simulink model "TuneWall"  (R2025b)
settings: Solver=VariableStepAuto  StartTime=0.0  StopTime=3600*4  RelTol=1e-3
model workspace (MAT data in the model file):
  h_in = 1.419
  h_out = 3.859
  k_Block = 0.01
  k_concrete = 0.11
libraries: fl_lib x66, nesl_utility x19, SimscapeFluids_lib x8
(part 1 of 2)
settings Model: Creator=Windows  LastModifiedBy=acer

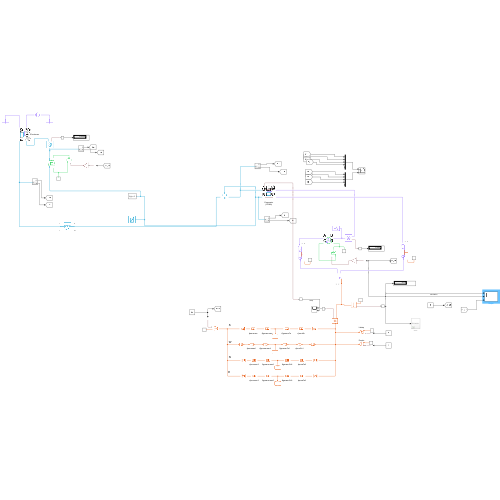
[thumbnail: Simulink's stored preview of the top-level diagram]
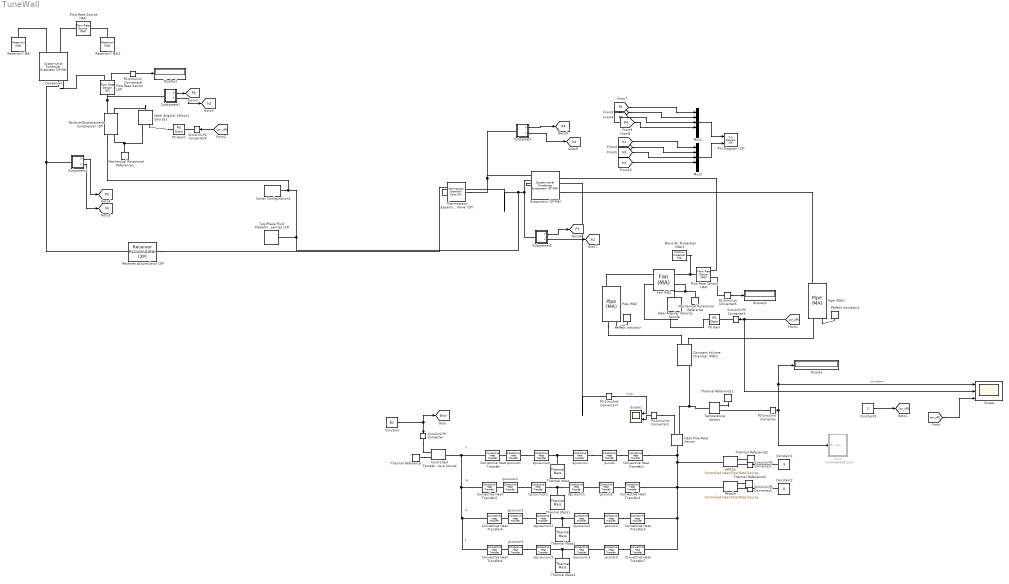
== system TuneWall ==
  note: S
  note: W
  note: N
  note: E
  Condenser : SimscapeFluids_lib/Heat Exchangers/Two-Phase Fluid - Moist Air/System-Level Condenser Evaporator (2P-MA)  flow_arrangement=fluids.heat_exchangers.enum.SystemLevelFlowArrangement2PMA.Counter  wall_thermal_mass=false  mass_wall=1 kg  cp_wall=490 J/(K*kg)  nominal_init_wall=true  T_wall_init=293.15 K  area_A1=0.01 m^2  area_B1=0.01 m^2  area_A2=0.01 m^2  area_B2=0.01 m^2  operating_condition_2P=fluids.heat_exchangers.enum.SystemLevelOperatingCondition2PMA.Condenser  mdot_nominal_2P=0.0142 kg/s  delta_p_nominal_2P=0.01 MPa  pressure_spec_cond_2P=fluids.heat_exchangers.enum.SystemLevelPressureSpecCondenser2P.InletPressure  pressure_spec_evap_2P=fluids.heat_exchangers.enum.SystemLevelPressureSpecEvaporator2P.InletPressure  p_in_nominal_2P=1.673 MPa  T_cond_nominal_2P=313.15 K  T_evap_nominal_2P=243.15 K  inlet_spec_2P=fluids.heat_exchangers.enum.SystemLevelInletSpec2P.Enthalpy  T_in_nominal_2P=333.15 K  h_in_nominal_2P=423.9 kJ/kg  x_in_nominal_2P=1  capacity_spec_2P=fluids.heat_exchangers.enum.SystemLevelCapacitySpec.HeatTransfer  Q_nominal=2.404 kW  outlet_spec_cond_2P=fluids.heat_exchangers.enum.SystemLevelOutletSpecCondenser2P.Enthalpy  outlet_spec_evap_2P=fluids.heat_exchangers.enum.SystemLevelOutletSpecEvaporator2P.Enthalpy  delta_T_sub_nominal_2P=5 deltaK  delta_T_sup_nominal_2P=5 deltaK  h_out_nominal_2P=250 kJ/kg  x_out_nominal_2P=0  volume_2P=0.001 m^3  nominal_init_2P=true  energy_spec_2P=foundation.enum.energy_spec.enthalpy  p_init_2P=0.101325 MPa  T_init_2P=293.15 K  x_init_2P=0.5  alpha_init_2P=0.5  h_init_2P=1500 kJ/kg  u_init_2P=1500 kJ/kg  mdot_nominal_MA=1 kg/s  delta_p_nominal_MA=0.001 MPa  p_in_nominal_MA=0.101325 MPa  T_in_nominal_MA=293.15 K  inlet_humidity_spec_MA=foundation.enum.HumiditySpec.RelativeHumidity  RH_in_nominal_MA=0.5  x_w_in_nominal_MA=0.01  y_w_in_nominal_MA=0.01  HR_in_nominal_MA=0.01  Tw_in_nominal_MA=287 K  inlet_trace_gas_spec_MA=foundation.enum.trace_gas_spec.mass_fraction  x_g_in_nominal_MA=0.001  y_g_in_nominal_MA=0.001  volume_MA=0.1 m^3  nominal_init_MA=true  p_init_MA=0.101325 MPa  T_init_MA=293.15 K  humidity_spec_MA=foundation.enum.HumiditySpec.RelativeHumidity  RH_init_MA=0.5  x_w_init_MA=0.01  y_w_init_MA=0.01  HR_init_MA=0.01  Tw_init_MA=287 K  trace_gas_spec_MA=foundation.enum.trace_gas_spec.mass_fraction  x_g_init_MA=0.001  y_g_init_MA=0.001  r_d_init_MA=0  RH_ws_MA=1  time_constant_cond_MA=1e-3 s  time_constant_evap_MA=1e-3 s  fraction_entrained_MA=1  a_liq_2P=0.023  a_mix_2P=0.005  a_vap_2P=0.023  b_2P=0.8  c_2P=0.33  a_MA=0.023  b_MA=0.8  c_MA=0.33
      settings: InternalSimscapePortConfiguration="{\"Bottom\":[],\"Left\":[{\"id\":\"A1\",\"label\":\"A1\",\"type\":\"foundation.two_phase_fluid.two_phase_fluid\"},{\"id\":\"B1\",\"label\":\"B1\",\"type\":\"foundation.two_phase_fluid.two_phase_fluid\"}],\"Right\":[{\"id\":\"A2\",\"label\":\"A2\",\"type\":\"foundation.moist_air.moist_air\"},{\"id\":\"B2\",\"label\":\"B2\",\"type\":\"foundation.moist_air.moist_air\"}],\"Top\":[{\"id\":\"Q1\",\"label\":\"Q1\",\"type\":\"output\"},{\"id\":\"Q2\",\"label\":\"Q2\",\"type\":\"output\"},{\"id\":\"W\",\"label\":\"W\",\"type\":\"output\"}]}"
  Constant : Constant  Value=30
  Constant Volume Chamber (MA)2 : fl_lib/Moist Air/Elements/Constant Volume Chamber (MA)  volume=92.924 m^3  num_ports=foundation.enum.num_ports.two  area_A=0.01 m^2  area_B=0.01 m^2  area_C=0.01 m^2  area_D=0.01 m^2  RH_ws=1  time_constant_cond=1e-3 s  time_constant_evap=1e-3 s  fraction_entrained=1  moisture_trace_gas_source=foundation.enum.moisture_trace_gas_source.none  moisture_source_spec=foundation.enum.MoistureSourceSpec.WaterVapor  vapor_from_liquid=false  moisture_mass_flow=0 kg/s  moisture_temperature_spec=foundation.enum.temperature_spec.atmospheric  moisture_temperature=293.15 K  trace_gas_mass_flow=0 kg/s  trace_gas_temperature_spec=foundation.enum.temperature_spec.atmospheric  trace_gas_temperature=293.15 K  p_init=0.101325 MPa  p_init_priority=foundation.enum.Priority.High  T_init=273.15+30 K  T_init_priority=foundation.enum.Priority.High  humidity_spec=foundation.enum.HumiditySpec.RelativeHumidity  RH_init=0.6  RH_init_priority=foundation.enum.Priority.High  x_w_init=0.01  x_w_init_priority=foundation.enum.Priority.High  y_w_init=0.01  y_w_init_priority=foundation.enum.Priority.High  HR_init=0.01  HR_init_priority=foundation.enum.Priority.High  Tw_init=287 K  Tw_init_priority=foundation.enum.Priority.High  trace_gas_spec=foundation.enum.trace_gas_spec.mass_fraction  x_g_init=0.001  x_g_init_priority=foundation.enum.Priority.High  y_g_init=0.001  y_g_init_priority=foundation.enum.Priority.High  r_d_init=0  r_d_init_priority=foundation.enum.Priority.High
      settings: InternalSimscapePortConfiguration="{\"Bottom\":[],\"Left\":[{\"id\":\"A\",\"label\":\"A\",\"type\":\"foundation.moist_air.moist_air\"},{\"id\":\"B\",\"label\":\"B\",\"type\":\"foundation.moist_air.moist_air\"}],\"Right\":[{\"id\":\"W\",\"label\":\"W\",\"type\":\"output\"},{\"id\":\"F\",\"label\":\"F\",\"type\":\"output\"},{\"id\":\"H\",\"label\":\"H\",\"type\":\"foundation.thermal.thermal\"}],\"Top\":[]}"
  Constant1 : Constant  Value=3
  Constant2 : Constant  Value=0
  Constant3 : Constant
  Controlled Temperature Source : fl_lib/Thermal/Thermal Sources/Controlled Temperature Source
  Convective Heat Transfer : fl_lib/Thermal/Thermal Elements/Convective Heat Transfer  thermal_type=foundation.enum.constant_variable.constant  area=8.51*3 m^2  heat_tr_coeff=h_out W/(K*m^2)  min_heat_tr_coeff=1e-3 W/(K*m^2)  T_specify=off  T_priority=None  T=0 K  T_nominal_specify=off  T_nominal_value=1  T_nominal_unit=K  Q_specify=off  Q_priority=None  Q=0 W  Q_nominal_specify=off  Q_nominal_value=1  Q_nominal_unit=W
  Convective Heat Transfer1 : fl_lib/Thermal/Thermal Elements/Convective Heat Transfer  thermal_type=foundation.enum.constant_variable.constant  area=8.51*3 m^2  heat_tr_coeff=h_in W/(K*m^2)  min_heat_tr_coeff=1e-3 W/(K*m^2)  T_specify=off  T_priority=None  T=0 K  T_nominal_specify=off  T_nominal_value=1  T_nominal_unit=K  Q_specify=off  Q_priority=None  Q=0 W  Q_nominal_specify=off  Q_nominal_value=1  Q_nominal_unit=W
  Convective Heat Transfer2 : fl_lib/Thermal/Thermal Elements/Convective Heat Transfer  thermal_type=foundation.enum.constant_variable.constant  area=8.86*3 m^2  heat_tr_coeff=h_out W/(K*m^2)  min_heat_tr_coeff=1e-3 W/(K*m^2)  T_specify=off  T_priority=None  T=0 K  T_nominal_specify=off  T_nominal_value=1  T_nominal_unit=K  Q_specify=off  Q_priority=None  Q=0 W  Q_nominal_specify=off  Q_nominal_value=1  Q_nominal_unit=W
  Convective Heat Transfer3 : fl_lib/Thermal/Thermal Elements/Convective Heat Transfer  thermal_type=foundation.enum.constant_variable.constant  area=8.86*3 m^2  heat_tr_coeff=h_in W/(K*m^2)  min_heat_tr_coeff=1e-3 W/(K*m^2)  T_specify=off  T_priority=None  T=0 K  T_nominal_specify=off  T_nominal_value=1  T_nominal_unit=K  Q_specify=off  Q_priority=None  Q=0 W  Q_nominal_specify=off  Q_nominal_value=1  Q_nominal_unit=W
  Convective Heat Transfer4 : fl_lib/Thermal/Thermal Elements/Convective Heat Transfer  thermal_type=foundation.enum.constant_variable.constant  area=8.51*3 m^2  heat_tr_coeff=h_out W/(K*m^2)  min_heat_tr_coeff=1e-3 W/(K*m^2)  T_specify=off  T_priority=None  T=0 K  T_nominal_specify=off  T_nominal_value=1  T_nominal_unit=K  Q_specify=off  Q_priority=None  Q=0 W  Q_nominal_specify=off  Q_nominal_value=1  Q_nominal_unit=W
  Convective Heat Transfer5 : fl_lib/Thermal/Thermal Elements/Convective Heat Transfer  thermal_type=foundation.enum.constant_variable.constant  area=8.51*3 m^2  heat_tr_coeff=h_in W/(K*m^2)  min_heat_tr_coeff=1e-3 W/(K*m^2)  T_specify=off  T_priority=None  T=0 K  T_nominal_specify=off  T_nominal_value=1  T_nominal_unit=K  Q_specify=off  Q_priority=None  Q=0 W  Q_nominal_specify=off  Q_nominal_value=1  Q_nominal_unit=W
  Convective Heat Transfer6 : fl_lib/Thermal/Thermal Elements/Convective Heat Transfer  thermal_type=foundation.enum.constant_variable.constant  area=8.86*3 m^2  heat_tr_coeff=h_out W/(K*m^2)  min_heat_tr_coeff=1e-3 W/(K*m^2)  T_specify=off  T_priority=None  T=0 K  T_nominal_specify=off  T_nominal_value=1  T_nominal_unit=K  Q_specify=off  Q_priority=None  Q=0 W  Q_nominal_specify=off  Q_nominal_value=1  Q_nominal_unit=W
  Convective Heat Transfer7 : fl_lib/Thermal/Thermal Elements/Convective Heat Transfer  thermal_type=foundation.enum.constant_variable.constant  area=8.86*3 m^2  heat_tr_coeff=h_in W/(K*m^2)  min_heat_tr_coeff=1e-3 W/(K*m^2)  T_specify=off  T_priority=None  T=0 K  T_nominal_specify=off  T_nominal_value=1  T_nominal_unit=K  Q_specify=off  Q_priority=None  Q=0 W  Q_nominal_specify=off  Q_nominal_value=1  Q_nominal_unit=W
  Display : Display
      settings: Decimation=3
  Display1 : Display
  Display2 : Display
  Evaporator (2P-MA) : SimscapeFluids_lib/Heat Exchangers/Two-Phase Fluid - Moist Air/System-Level Condenser Evaporator (2P-MA)  flow_arrangement=fluids.heat_exchangers.enum.SystemLevelFlowArrangement2PMA.Counter  wall_thermal_mass=false  mass_wall=1 kg  cp_wall=490 J/(K*kg)  nominal_init_wall=true  T_wall_init=293.15 K  area_A1=0.71 cm^2  area_B1=1.96 cm^2  area_A2=0.01 m^2  area_B2=0.01 m^2  operating_condition_2P=fluids.heat_exchangers.enum.SystemLevelOperatingCondition2PMA.Evaporator  mdot_nominal_2P=0.0142 kg/s  delta_p_nominal_2P=0.01 MPa  pressure_spec_cond_2P=fluids.heat_exchangers.enum.SystemLevelPressureSpecCondenser2P.InletPressure  pressure_spec_evap_2P=fluids.heat_exchangers.enum.SystemLevelPressureSpecEvaporator2P.InletPressure  p_in_nominal_2P=0.5806 MPa  T_cond_nominal_2P=313.15 K  T_evap_nominal_2P=243.15 K  inlet_spec_2P=fluids.heat_exchangers.enum.SystemLevelInletSpec2P.Enthalpy  T_in_nominal_2P=333.15 K  h_in_nominal_2P=253.3 kJ/kg  x_in_nominal_2P=1  capacity_spec_2P=fluids.heat_exchangers.enum.SystemLevelCapacitySpec.HeatTransfer  Q_nominal=2.31 kW  outlet_spec_cond_2P=fluids.heat_exchangers.enum.SystemLevelOutletSpecCondenser2P.Enthalpy  outlet_spec_evap_2P=fluids.heat_exchangers.enum.SystemLevelOutletSpecEvaporator2P.Enthalpy  delta_T_sub_nominal_2P=5 deltaK  delta_T_sup_nominal_2P=5 deltaK  h_out_nominal_2P=250 kJ/kg  x_out_nominal_2P=0  volume_2P=0.001 m^3  nominal_init_2P=true  energy_spec_2P=foundation.enum.energy_spec.enthalpy  p_init_2P=0.101325 MPa  T_init_2P=293.15 K  x_init_2P=0.5  alpha_init_2P=0.5  h_init_2P=1500 kJ/kg  u_init_2P=1500 kJ/kg  mdot_nominal_MA=1 kg/s  delta_p_nominal_MA=0.001 MPa  p_in_nominal_MA=0.101325 MPa  T_in_nominal_MA=29+273.15 K  inlet_humidity_spec_MA=foundation.enum.HumiditySpec.RelativeHumidity  RH_in_nominal_MA=0.5  x_w_in_nominal_MA=0.01  y_w_in_nominal_MA=0.01  HR_in_nominal_MA=0.01  Tw_in_nominal_MA=287 K  inlet_trace_gas_spec_MA=foundation.enum.trace_gas_spec.mass_fraction  x_g_in_nominal_MA=0.001  y_g_in_nominal_MA=0.001  volume_MA=0.1 m^3  nominal_init_MA=true  p_init_MA=0.101325 MPa  T_init_MA=293.15 K  humidity_spec_MA=foundation.enum.HumiditySpec.RelativeHumidity  RH_init_MA=0.5  x_w_init_MA=0.01  y_w_init_MA=0.01  HR_init_MA=0.01  Tw_init_MA=287 K  trace_gas_spec_MA=foundation.enum.trace_gas_spec.mass_fraction  x_g_init_MA=0.001  y_g_init_MA=0.001  r_d_init_MA=0  RH_ws_MA=1  time_constant_cond_MA=1e-3 s  time_constant_evap_MA=1e-3 s  fraction_entrained_MA=1  a_liq_2P=0.023  a_mix_2P=0.005  a_vap_2P=0.023  b_2P=0.8  c_2P=0.33  a_MA=0.023  b_MA=0.8  c_MA=0.33
      settings: InternalSimscapePortConfiguration="{\"Bottom\":[],\"Left\":[{\"id\":\"A1\",\"label\":\"A1\",\"type\":\"foundation.two_phase_fluid.two_phase_fluid\"},{\"id\":\"B1\",\"label\":\"B1\",\"type\":\"foundation.two_phase_fluid.two_phase_fluid\"}],\"Right\":[{\"id\":\"A2\",\"label\":\"A2\",\"type\":\"foundation.moist_air.moist_air\"},{\"id\":\"B2\",\"label\":\"B2\",\"type\":\"foundation.moist_air.moist_air\"}],\"Top\":[{\"id\":\"Q1\",\"label\":\"Q1\",\"type\":\"output\"},{\"id\":\"Q2\",\"label\":\"Q2\",\"type\":\"output\"},{\"id\":\"W\",\"label\":\"W\",\"type\":\"output\"}]}"
  Fan (MA) : SimscapeFluids_lib/Moist Air/Turbomachinery/Fan (MA)  fan_parameterization=fluids.moist_air.turbomachinery.enum.FanParameterization.Nominal  mechanical_power_spec=fluids.moist_air.turbomachinery.enum.FanMechanicalPowerSpec.Efficiency  flow_rate_nominal=0.38 m^3/s  pressure_nominal=5400 Pa  eta_nominal=1  power_nominal=1620 W  pressure_max=6400 Pa  flow_rate_max=0.4 m^3/s  omega_ref_nominal=1800 rpm  flow_rate_1D_TLU=[.0278, .0556, .0833, .111, .139, .167] m^3/s  pressure_1D_TLU=[6410, 6375, 6018, 5366, 4501, 3609] Pa  eta_1D_TLU=[.257, .394, .453, .47, .459, .415]  power_1D_TLU=[693, 900, 1107, 1267, 1363, 1452] W  omega_ref_1D=3000 rpm  rho_ref_1D=1.2 kg/m^3  omega_threshold_factor=1e-2  omega_dp_TLU=[2400; 3000; 3600] rpm  flow_rate_dp_TLU=[.0278, .0556, .0833, .111, .139, .167] m^3/s  pressure_dp_TLU=[4111, 4010, 3551, 2881, 2167, 1453; 6410, 6375, 6018, 5366, 4501, 3609; 9217, 9285, 9022, 8428, 7552, 6482] Pa  eta_dp_TLU=[.3, .434, .468, .459, .4, .3; .257, .394, .453, .47, .459, .415; .225, .359, .434, .461, .47, .459]  power_dp_TLU=[381, 514, 632, 697, 753, 809; 693, 900, 1107, 1267, 1363, 1452; 1139, 1438, 1732, 2029, 2233, 2358] W  rho_ref_dp=1.2 kg/m^3  omega_q_TLU=[2990; 3450; 3867] rpm  pressure_q_TLU=[31, 62, 93, 124] Pa  flow_rate_q_TLU=[.802, .759, .703, .611; .936, .902, .862, .81; 1.056, 1.027, .994, .956] m^3/s  eta_q_TLU=[.088, .162, .22, .261; .068, .128, .18, .222; .055, .105, .148, .188]  power_q_TLU=[283, 290, 297, 290; 427, 437, 445, 452; 595, 606, 625, 631] W  rho_ref_q=1.2 kg/m^3  diameter_ratio=1  mech_orientation=fluids.moist_air.turbomachinery.enum.FanMechanicalOrientation.Positive  area_A=0.01 m^2  area_B=0.01 m^2
      settings: InternalSimscapePortConfiguration="{\"Bottom\":[],\"Left\":[{\"id\":\"A\",\"label\":\"A\",\"type\":\"foundation.moist_air.moist_air\"},{\"id\":\"C\",\"label\":\"C\",\"type\":\"foundation.mechanical.rotational.rotational\"}],\"Right\":[{\"id\":\"B\",\"label\":\"B\",\"type\":\"foundation.moist_air.moist_air\"},{\"id\":\"R\",\"label\":\"R\",\"type\":\"foundation.mechanical.rotational.rotational\"}],\"Top\":[]}"
  Flow Rate Sensor (2P) : fl_lib/Two-Phase Fluid/Sensors/Flow Rate Sensor (2P)  mass_flow_measure=true  volumetric_flow_measure=false  energy_flow_measure=false
      settings: InternalSimscapePortConfiguration="{\"Bottom\":[],\"Left\":[{\"id\":\"A\",\"label\":\"A\",\"type\":\"foundation.two_phase_fluid.two_phase_fluid\"}],\"Right\":[{\"id\":\"B\",\"label\":\"B\",\"type\":\"foundation.two_phase_fluid.two_phase_fluid\"},{\"id\":\"M\",\"label\":\"M\",\"type\":\"output\"}],\"Top\":[]}"
  Flow Rate Sensor (MA) : fl_lib/Moist Air/Sensors/Flow Rate Sensor (MA)  mass_flow_measure=true  volumetric_flow_measure=false  volumetric_flow_conditions=foundation.enum.volumetric_flow_conditions.actual  p_std=0.101325 MPa  T_std=20 degC  RH_std=0.65  energy_flow_measure=false  vapor_flow_measure=false  gas_flow_measure=false  droplets_flow_measure=false
      settings: InternalSimscapePortConfiguration="{\"Bottom\":[],\"Left\":[{\"id\":\"A\",\"label\":\"A\",\"type\":\"foundation.moist_air.moist_air\"}],\"Right\":[{\"id\":\"B\",\"label\":\"B\",\"type\":\"foundation.moist_air.moist_air\"},{\"id\":\"M\",\"label\":\"M\",\"type\":\"output\"}],\"Top\":[]}"
  Flow Rate Source (MA) : fl_lib/Moist Air/Sources/Flow Rate Source (MA)  source_type=foundation.enum.constant_controlled.constant  flow_type=foundation.enum.mass_volumetric_flow.mass  mass_flow=1 kg/s  volumetric_flow=0 m^3/s  volumetric_flow_conditions=foundation.enum.volumetric_flow_conditions.actual  p_std=0.101325 MPa  T_std=20 degC  RH_std=0.65  power_spec=foundation.enum.power_spec.isentropic  area_A=0.01 m^2  area_B=0.01 m^2
      settings: InternalSimscapePortConfiguration="{\"Bottom\":[],\"Left\":[{\"id\":\"A\",\"label\":\"A\",\"type\":\"foundation.moist_air.moist_air\"}],\"Right\":[{\"id\":\"B\",\"label\":\"B\",\"type\":\"foundation.moist_air.moist_air\"}],\"Top\":[]}"
  Heat Flow Rate Sensor : fl_lib/Thermal/Thermal Sensors/Heat Flow Rate Sensor
  Ideal Angular Velocity Source : fl_lib/Mechanical/Mechanical Sources/Ideal Angular Velocity Source
  Ideal Angular Velocity Source1 : fl_lib/Mechanical/Mechanical Sources/Ideal Angular Velocity Source
  Labtop : fl_lib/Thermal/Thermal Sources/Controlled Heat Flow Rate Source
  Mechanical Rotational Reference : fl_lib/Mechanical/Rotational Elements/Mechanical Rotational Reference
  Mechanical Rotational Reference1 : fl_lib/Mechanical/Rotational Elements/Mechanical Rotational Reference
  Moist Air Properties (MA)1 : fl_lib/Moist Air/Utilities/Moist Air Properties (MA)  R_a=287.047 J/(K*kg)  T_TLU=[-56.55, -50 : 10 : -10, -5 : 1 : 5, 10 : 10 : 350]' degC  h_a_TLU=[342.414066793634; 349.003411914139; 359.061417476782; 369.117728274935; 379.173188407993; 389.228602960013; 394.256538873206; 395.262156814682; 396.26778682262; 397.27342967397; 398.279086145689; 399.284757014822; 400.290443058569; 401.296145054364; 402.301863779931; 403.307600013352; 404.313354533128; 409.342428711098; 419.402397945314; 429.465451846544; 439.532387826623; 449.604014793745; 459.68115297076; 469.764632657687; 479.855292205971; 489.953975419749; 500.06152856014; 510.178797098051; 520.306622336267; 530.445838000969; 540.597266885076; 550.761717610289; 560.939981561004; 571.132830031086; 581.341011613777; 591.565249855533; 601.806241186423; 612.064653132654; 622.341122810862; 632.636255698901; 642.95062467384; 653.284769304793; 663.639195385783; 674.014374692179; 684.410744943084; 694.828709951456; 705.268639943519; 715.730872029167; 726.215710805484; 736.723429076127; 747.254268670154; 757.808441344776] kJ/kg  mu_a_TLU=[14.2568884161326; 14.6140128551699; 15.151727785151; 15.6806860927178; 16.201235181264; 16.7137043838401; 16.9670072430524; 17.017438132541; 17.0677931537044; 17.1180726001803; 17.1682767640582; 17.2184059358881; 17.2684604046898; 17.318440457962; 17.3683463816913; 17.4181784603614; 17.467936976962; 17.7156359301048; 18.2056752419787; 18.6887904184394; 19.1652345249932; 19.6352479488881; 20.099059157425; 20.5568854116507; 21.008933436444; 21.4554000485251; 21.8964727442509; 22.3323302492491; 22.7631430320408; 23.1890737838183; 23.6102778665211; 24.0269037312887; 24.4390933092858; 24.8469823767971; 25.2507008963847; 25.6503733357905; 26.0461189661617; 26.438052141067; 26.8262825576728; 27.210915501349; 27.5920520748824; 27.969789413389; 28.3442208859359; 28.7154362848061; 29.0835220032714; 29.4485612026716; 29.8106339695395; 30.169817463453; 30.5261860562487; 30.8798114631771; 31.2307628665438; 31.5791070323335] s*uPa  k_a_TLU=[19.8808491891482; 20.4162457047568; 21.2248745869044; 22.0232455041378; 22.8117316528767; 23.59069155438; 23.9767077285082; 24.0536401764626; 24.130482853517; 24.2072360894785; 24.2839002127411; 24.3604755502875; 24.4369624276914; 24.5133611691197; 24.5896720973349; 24.6658955336975; 24.7420317981691; 25.1214166432482; 25.8738284673185; 26.6180151791963; 27.3542675863918; 28.0828636150405; 28.8040688184917; 29.5181369069754; 30.2253102842368; 30.9258205811167; 31.6198891790667; 32.307727718801; 32.989538590917; 33.6655154065126; 34.3358434467079; 35.0007000906151; 35.6602552217624; 36.314671613305; 36.9641052925838; 37.6087058857479; 38.2486169432557; 38.8839762471259; 39.5149161008418; 40.1415636028127; 40.7640409042923; 41.3824654526272; 41.9969502206863; 42.6076039232795; 43.2145312213471; 43.8178329146528; 44.4176061236819; 45.0139444614019; 45.6069381955058; 46.1966744017242; 46.7832371087507; 47.3667074352967] mW/(K*m)  p_min=1 kPa  p_max=inf MPa  T_min=-56.55 degC  T_max=350 degC  properties_range_check=simscape.enum.assert.action.error  p_atm=0.101325 MPa  T_atm=20 degC  enable_droplets=false  R_w=461.523 J/(K*kg)  p_ws_TLU=[1.71168953425982e-06; 3.93770601979424e-06; 1.28411717710344e-05; 3.80051394873809e-05; .00010323902900209; .000259873810798063; .000401741022116384; .000437454836117844; .000476040820618202; .000517704666185737; .000562664883741207; .000611212677444345; .000657085634113763; .000705985593917791; .00075808051438111; .000813548355379396; .000872575113841924; .00122819910164487; .00233931836947519; .00424697076171126; .00738493802968097; .012351945812707; .0199464343236764; .0312009300307261; .0474144740241604; .0701817658485933; .101417996663294; .143378712947169; .198674420476403; .270279976781692; .361539099388177; .476164537971214; .618234621423587; .792187006980199; 1.00281053608169; 1.25523615516845; 1.55492790046272; 1.90767499353199; 2.31958617020155; 2.79708749692822; 3.34692514426746; 3.97617493064794; 4.69226099229504; 5.50298678300951; 6.41658290952841; 7.44177834442093; 8.58790494083256; 9.86505121117553; 11.284292927457; 12.8580516000122; 14.6006773719404; 16.5294151389953] MPa  h_w_vap_TLU=[2836.88241275372; 2837.81392500514; 2838.63937175807; 2838.7309929628; 2838.06905313927; 2836.62597341095; 2835.60023952573; 2835.37006381376; 2835.13143158077; 2834.88429145066; 2834.62859062897; 2500.93420564316; 2498.55452890293; 2496.17317793437; 2493.7941260618; 2491.41713708944; 2489.04199020767; 2477.18706302224; 2453.51925941961; 2429.81122987564; 2405.97728678685; 2381.94712654051; 2357.65452030374; 2333.03120800924; 2308.00352809267; 2282.49062771796; 2256.40372152657; 2229.64615315163; 2202.11407337172; 2173.6974807639; 2144.28128268553; 2113.74600964951; 2081.9678834089; 2048.81807129851; 2014.16109962579; 1977.85249331179; 1939.73572816654; 1899.63852389863; 1857.36838273035; 1812.70710332357; 1765.4037880462; 1715.16561416478; 1661.64526339623; 1604.4232249434; 1542.98206457018; 1476.66790089115; 1404.63083498414; 1325.72875296442; 1238.36212284382; 1140.16281350074; 1027.31658328826; 892.746804215825] kJ/kg  h_w_TLU=[2396.53078650168; 2408.65722023252; 2427.16766028467; 2445.66624034104; 2464.1379798878; 2482.5594701893; 2491.7412703989; 2493.57467660537; 2495.40699233755; 2497.23816944599; 2499.06815833272; 2500.89261781717; 2502.73123919979; 2504.56496564907; 2506.39800457704; 2508.23033644628; 2510.06194120626; 2519.20831890725; 2537.43340437276; 2555.54520329515; 2573.51032237465; 2591.28888786817; 2608.83487221908; 2626.09640083333; 2643.01588134754; 2659.53001419864; 2675.5827869577; 2696.18462565746; 2716.49989554204; 2736.6235211014; 2756.61216047677; 2776.50561774616; 2796.33378923373; 2816.11979584021; 2835.88181424959; 2855.6343057571; 2875.38889328914; 2895.15500578618; 2914.94035966265; 2934.75132291939; 2954.59319332093; 2974.47041287496; 2994.38673461102; 3014.34535330297; 3034.34900869544; 3054.40006758361; 3074.50058949656; 3094.65237956705; 3114.85703131193; 3135.11596141057; 3155.43043809331; 3175.80160439414] kJ/kg  mu_w_TLU=[6.9886414857741; 7.21462000349698; 7.55962537406626; 7.90463074463554; 8.24963611520482; 8.5946414857741; 8.76714417105874; 8.80164470811567; 8.8361452451726; 8.87064578222952; 8.90514631928645; 8.93964685634338; 8.97414739340031; 9.00294911497154; 9.0318980288863; 9.06099135942002; 9.09022638806001; 9.23843559844524; 9.5440595677542; 9.86015858692705; 10.1848429274122; 10.5164578096049; 10.8535319382781; 11.1947482575333; 11.5389294976352; 11.8850331780701; 12.2322493177351; 12.6188533568459; 13.0082793358938; 13.4003380262893; 13.7948421428098; 14.1916095618232; 14.590464747099; 14.9912394314964; 15.3937729006119; 15.7979120385447; 16.203511226482; 16.610432150303; 17.0185435533718; 17.4277209582061; 17.8378463726577; 18.2488079909412; 18.6604998963166; 19.0728217698535; 19.485678608085; 19.8989804512625; 20.3126421231677; 20.7265829829225; 21.1407266888906; 21.5550009745266; 21.969337435876; 22.3836713303269] s*uPa  k_w_TLU=[12.4916816538045; 12.9847788176262; 13.737598915064; 14.4904190125018; 15.2432391099396; 15.9960592073774; 16.3724692560963; 16.4477512658401; 16.5230332755839; 16.5983152853277; 16.6735972950715; 16.7488793048152; 16.824161314559; 16.8886088206517; 16.9532779906513; 17.0181691764255; 17.083282769915; 17.4122036181723; 18.0870861656185; 18.7855813517187; 19.5093466408385; 20.2607864040347; 21.0430876297671; 21.8602068151121; 22.7168164077153; 23.6182141540994; 24.5698636875305; 25.4024944426483; 26.2458938647479; 27.1009155051916; 27.968142896353; 28.8479507975112; 29.7405485790829; 30.646029672269; 31.5643932662527; 32.4955693285114; 33.4394360046859; 34.3958329885356; 35.3645718140131; 36.3454437886179; 37.3382261129791; 38.3426866012072; 39.3585873185985; 40.3856873794121; 41.4237450915028; 42.4725195920623; 43.5317720862424; 44.6012667755489; 45.6807715437344; 46.7700584531355; 47.8689040929333; 48.9770898119082] mW/(K*m)  D_w=25 mm^2/s  trace_gas_model=foundation.enum.trace_gas_model.none  R_g=188.923 J/(K*kg)  h_g_TLU=[439.555216276024; 444.670268214299; 452.538618857965; 460.487124266174; 468.522588773143; 476.64941595933; 480.747985385885; 481.570543185868; 482.394052396612; 483.218514286302; 484.043930026094; 484.87030069324; 485.697627274149; 486.525910667382; 487.355151686572; 488.185351063277; 489.016509449741; 493.186704132078; 501.599194941473; 510.107689945701; 518.711611059603; 527.410026767716; 536.20176474847; 545.085474167968; 554.059675464379; 563.122805439004; 572.273250917104; 581.509372969931; 590.829525041787; 600.232066635428; 609.715373504524; 619.277845094572; 628.91790983254; 638.634028741375; 648.424697754692; 658.288449028076; 668.22385148184; 678.229510761734; 688.30406876583; 698.446202855373; 708.654624842952; 718.928079831753; 729.265344963773; 739.665228122078; 750.126566621791; 760.648225916092; 771.229098336723; 781.86810188302; 792.564179069104; 803.316295835373; 814.123440527678; 824.984622945405] kJ/kg  mu_g_TLU=[10.9386626034033; 11.2618160869372; 11.7542862475187; 12.2454955799777; 12.7352208796158; 13.2232325321233; 13.4665248390743; 13.5151226761166; 13.5636997995993; 13.6122559954699; 13.6607910510226; 13.709304754931; 13.757796897279; 13.8062672695897; 13.8547156648526; 13.9031418775498; 13.9515457036801; 14.1932220047332; 14.6747828595747; 15.153802214283; 15.6301123398299; 16.1035631756244; 16.574022106427; 17.0413733976215; 17.5055174102327; 17.9663696812767; 18.4238599299346; 18.8779310322956; 19.3285379947687; 19.7756469471288; 20.2192341695255; 20.6592851629269; 21.0957937689132; 21.5287613421341; 21.9581959768344; 22.3841117874779; 22.8065282425078; 23.2254695495877; 23.6409640901974; 24.0530439011453; 24.4617442003854; 24.8671029544344; 25.269160484669; 25.6679591098169; 26.0635428220247; 26.4559569939835; 26.8452481147025; 27.2314635516519; 27.6146513371198; 27.9948599767665; 28.3721382784874; 28.74653519983] s*uPa  k_g_TLU=[10.7373095949238; 11.1772934980884; 11.862915506018; 12.5638333280734; 13.2785475592421; 14.005722199619; 14.3736017704762; 14.4475028211958; 14.5215096973787; 14.5956213250986; 14.6698366403414; 14.7441545888563; 14.8185741260114; 14.8930942166532; 14.9677138349692; 15.0424319643548; 15.1172475972825; 15.4927536712633; 16.2505237772467; 17.0165521650722; 17.7899991951805; 18.5700903932503; 19.3561099002839; 20.1473949639617; 20.9433312278214; 21.7433486448307; 22.5469178892132; 23.3535471729555; 24.1627793965491; 24.9741895799701; 25.7873825314493; 26.6019907190427; 27.4176723115859; 28.2341093347412; 29.0510055857402; 29.8680879651392; 30.6851034165693; 31.5018116707882; 32.3179924018673; 33.1334410491403; 33.9479677779769; 34.7613965127281; 35.5735640361829; 36.3843191504339; 37.1935218945334; 38.0010428147395; 38.80676228352; 39.6105698638057; 40.412363715274; 41.2120500397018; 42.0095425626597; 42.8047620490288] mW/(K*m)  D_g=16 mm^2/s
  Mux1 : Mux  Inputs=5
  Mux2 : Mux  Inputs=5
  P-H Diagram (2P) : SimscapeFluids_lib/Two-Phase Fluid/Utilities/P-H Diagram (2P)  p_unit=MPa  h_unit=kJ/kg
  PS Gain : fl_lib/Physical Signals/Functions/PS Gain  gain=1800 rpm
  PS Gain1 : fl_lib/Physical Signals/Functions/PS Gain  gain=1000 rpm
  PS-Simulink Converter : nesl_utility/PS-Simulink Converter  PhysicalDomain=network_engine_domain  SubClassName=ps_output  LeftPortType=input  RightPortType=output  PseudoPeriodic=off  Frequencies=[]  VectorFormat=inherit  Unit=degC  AffineConversion=on
  PS-Simulink Converter1 : nesl_utility/PS-Simulink Converter  PhysicalDomain=network_engine_domain  SubClassName=ps_output  LeftPortType=input  RightPortType=output  PseudoPeriodic=off  Frequencies=[]  VectorFormat=inherit  Unit=kW  AffineConversion=on
  PS-Simulink Converter6 : nesl_utility/PS-Simulink Converter  PhysicalDomain=network_engine_domain  SubClassName=ps_output  LeftPortType=input  RightPortType=output  PseudoPeriodic=off  Frequencies=[]  VectorFormat=inherit  Unit=inherit  AffineConversion=off
  PS-Simulink Converter7 : nesl_utility/PS-Simulink Converter  PhysicalDomain=network_engine_domain  SubClassName=ps_output  LeftPortType=input  RightPortType=output  PseudoPeriodic=off  Frequencies=[]  VectorFormat=inherit  Unit=kW  AffineConversion=on
  PS-Simulink Converter8 : nesl_utility/PS-Simulink Converter  PhysicalDomain=network_engine_domain  SubClassName=ps_output  LeftPortType=input  RightPortType=output  PseudoPeriodic=off  Frequencies=[]  VectorFormat=inherit  Unit=inherit  AffineConversion=off
  People : fl_lib/Thermal/Thermal Sources/Controlled Heat Flow Rate Source
  Perfect Insulator : fl_lib/Thermal/Thermal Elements/Perfect Insulator  T_specify=off  T_priority=None  T=293.15 K  T_nominal_specify=off  T_nominal_value=1  T_nominal_unit=K
  Perfect Insulator1 : fl_lib/Thermal/Thermal Elements/Perfect Insulator  T_specify=off  T_priority=None  T=293.15 K  T_nominal_specify=off  T_nominal_value=1  T_nominal_unit=K
  Pipe (MA) : fl_lib/Moist Air/Elements/Pipe (MA)  length=5 m  area=0.01 m^2  Dh=0.1 m  length_add=0.1 m  roughness=15e-6 m  Re_lam=2000  Re_tur=4000  shape_factor=64  Nu_lam=3.66  wall_condensation=false  RH_ws=1  time_constant_cond=1e-3 s  time_constant_evap=1e-3 s  fraction_entrained=1  moisture_trace_gas_source=foundation.enum.moisture_trace_gas_source.none  moisture_source_spec=foundation.enum.MoistureSourceSpec.WaterVapor  vapor_from_liquid=false  moisture_mass_flow=0 kg/s  moisture_temperature_spec=foundation.enum.temperature_spec.atmospheric  moisture_temperature=293.15 K  trace_gas_mass_flow=0 kg/s  trace_gas_temperature_spec=foundation.enum.temperature_spec.atmospheric  trace_gas_temperature=293.15 K  p_init=0.101325 MPa  p_init_priority=foundation.enum.Priority.High  T_init=293.15 K  T_init_priority=foundation.enum.Priority.High  humidity_spec=foundation.enum.HumiditySpec.RelativeHumidity  RH_init=0.5  RH_init_priority=foundation.enum.Priority.High  x_w_init=0.01  x_w_init_priority=foundation.enum.Priority.High  y_w_init=0.01  y_w_init_priority=foundation.enum.Priority.High  HR_init=0.01  HR_init_priority=foundation.enum.Priority.High  Tw_init=287 K  Tw_init_priority=foundation.enum.Priority.High  trace_gas_spec=foundation.enum.trace_gas_spec.mass_fraction  x_g_init=0.001  x_g_init_priority=foundation.enum.Priority.High  y_g_init=0.001  y_g_init_priority=foundation.enum.Priority.High  r_d_init=0  r_d_init_priority=foundation.enum.Priority.High
  Pipe (MA)1 : fl_lib/Moist Air/Elements/Pipe (MA)  length=5 m  area=0.01 m^2  Dh=0.1 m  length_add=0.1 m  roughness=15e-6 m  Re_lam=2000  Re_tur=4000  shape_factor=64  Nu_lam=3.66  wall_condensation=false  RH_ws=1  time_constant_cond=1e-3 s  time_constant_evap=1e-3 s  fraction_entrained=1  moisture_trace_gas_source=foundation.enum.moisture_trace_gas_source.none  moisture_source_spec=foundation.enum.MoistureSourceSpec.WaterVapor  vapor_from_liquid=false  moisture_mass_flow=0 kg/s  moisture_temperature_spec=foundation.enum.temperature_spec.atmospheric  moisture_temperature=293.15 K  trace_gas_mass_flow=0 kg/s  trace_gas_temperature_spec=foundation.enum.temperature_spec.atmospheric  trace_gas_temperature=293.15 K  p_init=0.101325 MPa  p_init_priority=foundation.enum.Priority.High  T_init=293.15 K  T_init_priority=foundation.enum.Priority.High  humidity_spec=foundation.enum.HumiditySpec.RelativeHumidity  RH_init=0.5  RH_init_priority=foundation.enum.Priority.High  x_w_init=0.01  x_w_init_priority=foundation.enum.Priority.High  y_w_init=0.01  y_w_init_priority=foundation.enum.Priority.High  HR_init=0.01  HR_init_priority=foundation.enum.Priority.High  Tw_init=287 K  Tw_init_priority=foundation.enum.Priority.High  trace_gas_spec=foundation.enum.trace_gas_spec.mass_fraction  x_g_init=0.001  x_g_init_priority=foundation.enum.Priority.High  y_g_init=0.001  y_g_init_priority=foundation.enum.Priority.High  r_d_init=0  r_d_init_priority=foundation.enum.Priority.High
  Positive-Displacement Compressor (2P) : SimscapeFluids_lib/Two-Phase Fluid/Fluid Machines/Positive-Displacement Compressor (2P)  dispSpec=fluids.two_phase_fluid.fluid_machines.enum.DisplacementSpecification.Displacement  v_disp=40 cm^3/rev  mdot_nom=0.01 kg/s  omega_nom=1000 rpm  efficiencySpec=fluids.two_phase_fluid.fluid_machines.enum.VolumetricEfficiencyParameterization.Analytical  thermodynamicModelSpec=fluids.two_phase_fluid.fluid_machines.enum.ThermodynamicModel.Polytropic  n=1.25  eta_isen=0.65  eta_isen_TLU=[.95, .9, .85, .8, .75; .925, .875, .825, .775, .725; .875, .825, .775, .725, .675; .75, .7, .65, .6, .55]  eta_vol_nom=0.95  pr_TLU=[2, 4, 6, 8]  omega_TLU=[800, 1500, 2800, 3300, 4000] rpm  eta_vol_TLU=[.95, .9, .85, .8, .75; .925, .875, .825, .775, .725; .875, .825, .775, .725, .675; .75, .7, .65, .6, .55]  nominalSpec=fluids.two_phase_fluid.fluid_machines.enum.NominalConditionsSpecification.Pressure  pr_nom=2.88  p_in_nom=0.101325 MPa  T_in_nom=373.15 K  T_evap_nom=373.15 K  T_cond_nom=398.15 K  delta_T_nom=10 deltaK  mechanical_efficiency=0.9  area_A=0.01 m^2  area_B=0.01 m^2  VaporCheck=simscape.enum.assert.action.warn
      settings: InternalSimscapePortConfiguration="{\"Bottom\":[],\"Left\":[{\"id\":\"A\",\"label\":\"A\",\"type\":\"foundation.two_phase_fluid.two_phase_fluid\"},{\"id\":\"C\",\"label\":\"C\",\"type\":\"foundation.mechanical.rotational.rotational\"}],\"Right\":[{\"id\":\"B\",\"label\":\"B\",\"type\":\"foundation.two_phase_fluid.two_phase_fluid\"},{\"id\":\"R\",\"label\":\"R\",\"type\":\"foundation.mechanical.rotational.rotational\"}],\"Top\":[]}"
  Receiver Accumulator (2P) : SimscapeFluids_lib/Two-Phase Fluid/Tanks & Accumulators/Receiver Accumulator (2P)  volume=1 m^3  tank_area=0.5 m^2  area_AV=0.01 m^2  area_BV=0.01 m^2  area_AL=0.01 m^2  area_BL=0.01 m^2  V_frac_liq_error=simscape.enum.assert.action.none  V_frac_liq_min=0.05  V_frac_liq_max=0.95  V_frac_smooth=0.05  p_crit_error=simscape.enum.assert.action.error  hc_vap=20 W/(K*m^2)  hc_liq=100 W/(K*m^2)  p_init=1.673 MPa  fraction_spec=fluids.two_phase_fluid.tanks_accumulators.enum.LiquidFractionSpec.Volume  M_frac_liq_init=0.5  V_frac_liq_init=0.5  saturated_init=true  energy_spec=fluids.two_phase_fluid.tanks_accumulators.enum.EnergySpec.SubcoolingSuperheating  delta_T_sub_init=5 deltaK  delta_T_sup_init=5 deltaK  T_liq_init=368.15 K  T_vap_init=378.15 K  h_liq_init=400 kJ/kg  h_vap_init=2700 kJ/kg  u_liq_init=400 kJ/kg  u_vap_init=2700 kJ/kg  tau_vap_cond=0.1 s
      settings: InternalSimscapePortConfiguration="{\"Bottom\":[],\"Left\":[{\"id\":\"AV\",\"label\":\"AV\",\"type\":\"foundation.two_phase_fluid.two_phase_fluid\"},{\"id\":\"AL\",\"label\":\"AL\",\"type\":\"foundation.two_phase_fluid.two_phase_fluid\"},{\"id\":\"H\",\"label\":\"H\",\"type\":\"foundation.thermal.thermal\"}],\"Right\":[{\"id\":\"BV\",\"label\":\"BV\",\"type\":\"foundation.two_phase_fluid.two_phase_fluid\"},{\"id\":\"BL\",\"label\":\"BL\",\"type\":\"foundation.two_phase_fluid.two_phase_fluid\"},{\"id\":\"L\",\"label\":\"L\",\"type\":\"output\"}],\"Top\":[]}"
  Reservoir (MA) : fl_lib/Moist Air/Elements/Reservoir (MA)  pressure_input=false  pressure_spec=foundation.enum.pressure_spec.atmospheric  reservoir_pressure=0.101325 MPa  temperature_input=false  temperature_spec=foundation.enum.temperature_spec.atmospheric  reservoir_temperature=293.15 K  humidity_input=false  humidity_spec=foundation.enum.HumiditySpec.RelativeHumidity  reservoir_RH=0.5  reservoir_x_w=0.01  reservoir_y_w=0.01  reservoir_HR=0.01  reservoir_Tw=287 K  trace_gas_input=false  trace_gas_spec=foundation.enum.trace_gas_spec.mass_fraction  reservoir_x_g=0.001  reservoir_y_g=0.001  water_droplets_input=false  reservoir_r_d=0  RH_ws=1  area_A=0.01 m^2  input_error_spec=foundation.enum.input_range_error.warn
  Reservoir (MA)1 : fl_lib/Moist Air/Elements/Reservoir (MA)  pressure_input=false  pressure_spec=foundation.enum.pressure_spec.atmospheric  reservoir_pressure=0.101325 MPa  temperature_input=false  temperature_spec=foundation.enum.temperature_spec.atmospheric  reservoir_temperature=293.15 K  humidity_input=false  humidity_spec=foundation.enum.HumiditySpec.RelativeHumidity  reservoir_RH=0.5  reservoir_x_w=0.01  reservoir_y_w=0.01  reservoir_HR=0.01  reservoir_Tw=287 K  trace_gas_input=false  trace_gas_spec=foundation.enum.trace_gas_spec.mass_fraction  reservoir_x_g=0.001  reservoir_y_g=0.001  water_droplets_input=false  reservoir_r_d=0  RH_ws=1  area_A=0.01 m^2  input_error_spec=foundation.enum.input_range_error.warn
  Scope : Scope  NumInputPorts=3
      settings: ActiveDisplayYMinimum=-6.42685143301012  ActiveDisplayYMaximum=34.047427937001125  DataLoggingVariableName=ScopeData2
  Scope1 : Scope  NumInputPorts=2
      settings: ActiveDisplayYMinimum=0.96283204895950791  ActiveDisplayYMaximum=2.8874567998920733
  Simulink-PS Converter : nesl_utility/Simulink-PS Converter  PhysicalDomain=network_engine_domain  SubClassName=ps_input  LeftPortType=input  RightPortType=output  PseudoPeriodic=off  Frequencies=[]  NoiseDistribution=none  NoiseParameters=[]  Unit=degC  AffineConversion=on  FilteringAndDerivatives=provide  SimscapeFilterOrder=1  InputFilterTimeConstant=0.001  UdotUserProvided=0
  Simulink-PS Converter{1..4} (4 alike) : nesl_utility/Simulink-PS Converter  PhysicalDomain=network_engine_domain  SubClassName=ps_input  LeftPortType=input  RightPortType=output  PseudoPeriodic=off  Frequencies=[]  NoiseDistribution=none  NoiseParameters=[]  Unit=1  AffineConversion=off  FilteringAndDerivatives=provide  SimscapeFilterOrder=1  InputFilterTimeConstant=0.001  UdotUserProvided=0
  Solver Configuration1 : nesl_utility/Solver Configuration  PhysicalDomain=network_engine_domain  SubClassName=solver  LeftPortType=input  RightPortType=generic  Tones=[]  Harmonics=[]  SimulateNoise=off  Profile=off  UseLocalSampling=off  EnableSwitchedLinearOptims=on  FrequencyDomain=off  UseCCode=off  RelTol=0.001  AbsTol=0.001  MinStep=1e-09  ToWorkspace=off  RevertToSquareIcSolve=off  NumHomotopyIterations=100  PhasorMode=off  PhasorModeNumHarmonics=1  ConsistencySolver=NEWTON_XTOL_AFTER_FTOL  IndexReductionMethod=DerivativeReplacement  DoDC=off  ResidualTolerance=1e-09  ConsistencyTolSource=GLOBAL  ConsistencyAbsTol=0.001  ConsistencyRelTol=0.001  ConsistencyTolFactor=0.001  UseLocalSolver=off  LocalSolverChoice=NE_BACKWARD_EULER_ADVANCER  ResolveIndetEquations=on  FunctionEvalNumThread=1  LocalSolverSampleTime=0.001  DoFixedCost=off  MaxNonlinIter=3  MaxModeIter=2  ComputeImpulses=off  ImpulseIterations=2  LinearAlgebra=auto  LinearAlgebraNumThread=0  EquationFormulation=NE_TIME_EF  DelaysMemoryBudget=1024  AutomaticFiltering=on  FilteringTimeConstant=0.001  PartitionStorageMethod=AS_NEEDED  PartitionMemoryBudget=1024  PartitionMethod=ROBUST  MultibodyUseLocalSolver=off  MultibodyLocalSolverChoice=ODE1  MultibodyLocalSolverSampleTime=0.001
  Subsystem : Subsystem
  Subsystem1 : Subsystem
  Subsystem2 : Subsystem
  Subsystem3 : Subsystem
  Temperature Sensor : fl_lib/Thermal/Thermal Sensors/Temperature Sensor  temperature_measure=foundation.enum.MeasurementReference.difference
  Thermal Mass : fl_lib/Thermal/Thermal Elements/Thermal Mass  mass_type=foundation.enum.constant_variable.constant  mass=(8.51*3*0.2)*620 kg  sp_heat=840 J/(K*kg)  mass_min=1e-6 kg  num_ports=foundation.enum.numPorts2.one  m_specify=off  m_priority=High  m=1 kg  m_nominal_specify=off  m_nominal_value=1  m_nominal_unit=kg  T_specify=off  T_priority=High  T=273.15+29 K  T_nominal_specify=off  T_nominal_value=1  T_nominal_unit=K  Q_specify=off  Q_priority=None  Q=0 W  Q_nominal_specify=off  Q_nominal_value=1  Q_nominal_unit=W
  Thermal Mass1 : fl_lib/Thermal/Thermal Elements/Thermal Mass  mass_type=foundation.enum.constant_variable.constant  mass=(8.86*3*0.2)*620 kg  sp_heat=840 J/(K*kg)  mass_min=1e-6 kg  num_ports=foundation.enum.numPorts2.one  m_specify=off  m_priority=High  m=1 kg  m_nominal_specify=off  m_nominal_value=1  m_nominal_unit=kg  T_specify=off  T_priority=High  T=300 K  T_nominal_specify=off  T_nominal_value=25+273.15  T_nominal_unit=K  Q_specify=off  Q_priority=None  Q=0 W  Q_nominal_specify=off  Q_nominal_value=1  Q_nominal_unit=W
  Thermal Mass2 : fl_lib/Thermal/Thermal Elements/Thermal Mass  mass_type=foundation.enum.constant_variable.constant  mass=(8.51*3*0.2)*620 kg  sp_heat=840 J/(K*kg)  mass_min=1e-6 kg  num_ports=foundation.enum.numPorts2.one  m_specify=off  m_priority=High  m=1 kg  m_nominal_specify=off  m_nominal_value=1  m_nominal_unit=kg  T_specify=off  T_priority=High  T=300 K  T_nominal_specify=off  T_nominal_value=25+273.15  T_nominal_unit=K  Q_specify=off  Q_priority=None  Q=0 W  Q_nominal_specify=off  Q_nominal_value=1  Q_nominal_unit=W
  Thermal Mass3 : fl_lib/Thermal/Thermal Elements/Thermal Mass  mass_type=foundation.enum.constant_variable.constant  mass=(8.86*3*0.2)*620 kg  sp_heat=840 J/(K*kg)  mass_min=1e-6 kg  num_ports=foundation.enum.numPorts2.one  m_specify=off  m_priority=High  m=1 kg  m_nominal_specify=off  m_nominal_value=1  m_nominal_unit=kg  T_specify=off  T_priority=High  T=300 K  T_nominal_specify=off  T_nominal_value=25+273.15  T_nominal_unit=K  Q_specify=off  Q_priority=None  Q=0 W  Q_nominal_specify=off  Q_nominal_value=1  Q_nominal_unit=W
  Thermal Reference{,1..3} (4 alike) : fl_lib/Thermal/Thermal Elements/Thermal Reference
  Thermostatic Expansion Valve (2P) : SimscapeFluids_lib/Two-Phase Fluid/Valves & Orifices/Flow Control Valves/Thermostatic Expansion Valve (2P)  valve_parameterization=fluids.two_phase_fluid.valves_orifices.flow_control_valves.enum.ThermostaticExpansionValveParameterization.Nominal  capacity_spec=fluids.two_phase_fluid.valves_orifices.flow_control_valves.enum.ThermostaticExpansionValveCapacitySpec.HeatTransfer  Q_nominal=2.31 kW  Q_max=2.5 kW  mdot_nominal=0.005 kg/s  mdot_max=0.008 kg/s  pressure_spec=fluids.two_phase_fluid.valves_orifices.flow_control_valves.enum.ThermostaticExpansionValvePressureSpec.Pressure  p_cond_nominal=1.673 MPa  p_evap_nominal=0.5806 MPa  T_cond_nominal=333.15 K  T_evap_nominal=273.15 K  delta_T_sub=1 deltaK  delta_T_nominal=10 deltaK  delta_T_static=1 deltaK  mop=fluids.two_phase_fluid.valves_orifices.flow_control_valves.enum.ThermostaticExpansionValveMOP.Off  p_mop=0.5 MPa  T_mop=288.15 K  T_evap_out_TLU1=0 : 10 : 40 degC  p_bulb_TLU1=0.3 : 0.1 : 0.7 MPa  lift_TLU2=0 : 0.15 : 0.6 mm  p_evap_TLU2=0.3 : -0.05 : 0.1 MPa  lift_TLU3=0 : 0.15 : 0.6 mm  mdot_TLU3=[1e-7, 0.015 : 0.015 : 0.06] kg/s  p_cond_ref=2 MPa  p_evap_ref=0.3 MPa  T_evap_out_ref=0 degC  delta_T_sub_ref=5 deltaK  pressure_equalization=fluids.two_phase_fluid.valves_orifices.flow_control_valves.enum.ThermostaticExpansionValveEqualization.Internal  bulb_dynamics=false  tau_bulb=20 s  leakage_fraction=1e-6  smoothing_factor=0.01  B_lam=0.999  tau_x=0.1 s  area=0.01 m^2
      settings: InternalSimscapePortConfiguration="{\"Bottom\":[],\"Left\":[{\"id\":\"A\",\"label\":\"A\",\"type\":\"foundation.two_phase_fluid.two_phase_fluid\"}],\"Right\":[{\"id\":\"B\",\"label\":\"B\",\"type\":\"foundation.two_phase_fluid.two_phase_fluid\"}],\"Top\":[{\"id\":\"S\",\"label\":\"S\",\"type\":\"foundation.two_phase_fluid.two_phase_fluid\"}]}"
  Two-Phase Fluid Predefined Properties (2P) : SimscapeFluids_lib/Two-Phase Fluid/Utilities/Two-Phase Fluid Predefined Properties (2P)  fluid=fluids.two_phase_fluid.utilities.enum.Fluid.R22  p_atm=0.101325 MPa  properties_range_check=simscape.enum.assert.action.error  q_rev=0.01 Pa
  error : Subsystem  Commented=on
  ปูนฉาบนอก : fl_lib/Thermal/Thermal Elements/Conductive Heat Transfer  thermal_type=foundation.enum.ConstantVariableTabulated.Constant  wall_geometry=foundation.enum.ConductionWallGeometry.Planar  area=8.51*3 m^2  thickness=0.05 m  d_in=0.05 m  d_out=0.1 m  L=1 m  th_cond_min=10 W/(K*m)  th_cond=k_concrete W/(K*m)  th_cond_TLU=[413, 401, 392, 383, 371, 357, 342] W/(K*m)  temp_TLU=[200, 273, 400, 600, 800, 1000, 1200] K  T_specify=off  T_priority=None  T=0 K  T_nominal_specify=off  T_nominal_value=1  T_nominal_unit=K  Q_specify=off  Q_priority=None  Q=0 W  Q_nominal_specify=off  Q_nominal_value=1  Q_nominal_unit=W
  ปูนฉาบนอก1 : fl_lib/Thermal/Thermal Elements/Conductive Heat Transfer  thermal_type=foundation.enum.ConstantVariableTabulated.Constant  wall_geometry=foundation.enum.ConductionWallGeometry.Planar  area=8.86*3 m^2  thickness=0.01 m  d_in=0.05 m  d_out=0.1 m  L=1 m  th_cond_min=10 W/(K*m)  th_cond=k_concrete W/(K*m)  th_cond_TLU=[413, 401, 392, 383, 371, 357, 342] W/(K*m)  temp_TLU=[200, 273, 400, 600, 800, 1000, 1200] K  T_specify=off  T_priority=None  T=0 K  T_nominal_specify=off  T_nominal_value=1  T_nominal_unit=K  Q_specify=off  Q_priority=None  Q=0 W  Q_nominal_specify=off  Q_nominal_value=1  Q_nominal_unit=W
  ปูนฉาบนอก2 : fl_lib/Thermal/Thermal Elements/Conductive Heat Transfer  thermal_type=foundation.enum.ConstantVariableTabulated.Constant  wall_geometry=foundation.enum.ConductionWallGeometry.Planar  area=8.51*3 m^2  thickness=0.01 m  d_in=0.05 m  d_out=0.1 m  L=1 m  th_cond_min=10 W/(K*m)  th_cond=k_concrete W/(K*m)  th_cond_TLU=[413, 401, 392, 383, 371, 357, 342] W/(K*m)  temp_TLU=[200, 273, 400, 600, 800, 1000, 1200] K  T_specify=off  T_priority=None  T=0 K  T_nominal_specify=off  T_nominal_value=1  T_nominal_unit=K  Q_specify=off  Q_priority=None  Q=0 W  Q_nominal_specify=off  Q_nominal_value=1  Q_nominal_unit=W
  ปูนฉาบนอก3 : fl_lib/Thermal/Thermal Elements/Conductive Heat Transfer  thermal_type=foundation.enum.ConstantVariableTabulated.Constant  wall_geometry=foundation.enum.ConductionWallGeometry.Planar  area=8.86*3 m^2  thickness=0.01 m  d_in=0.05 m  d_out=0.1 m  L=1 m  th_cond_min=10 W/(K*m)  th_cond=k_concrete W/(K*m)  th_cond_TLU=[413, 401, 392, 383, 371, 357, 342] W/(K*m)  temp_TLU=[200, 273, 400, 600, 800, 1000, 1200] K  T_specify=off  T_priority=None  T=0 K  T_nominal_specify=off  T_nominal_value=1  T_nominal_unit=K  Q_specify=off  Q_priority=None  Q=0 W  Q_nominal_specify=off  Q_nominal_value=1  Q_nominal_unit=W
  ปูนฉาบใน : fl_lib/Thermal/Thermal Elements/Conductive Heat Transfer  thermal_type=foundation.enum.ConstantVariableTabulated.Constant  wall_geometry=foundation.enum.ConductionWallGeometry.Planar  area=8.51*3 m^2  thickness=0.05 m  d_in=0.05 m  d_out=0.1 m  L=1 m  th_cond_min=10 W/(K*m)  th_cond=k_concrete W/(K*m)  th_cond_TLU=[413, 401, 392, 383, 371, 357, 342] W/(K*m)  temp_TLU=[200, 273, 400, 600, 800, 1000, 1200] K  T_specify=off  T_priority=None  T=0 K  T_nominal_specify=off  T_nominal_value=1  T_nominal_unit=K  Q_specify=off  Q_priority=None  Q=0 W  Q_nominal_specify=off  Q_nominal_value=1  Q_nominal_unit=W
  ปูนฉาบใน1 : fl_lib/Thermal/Thermal Elements/Conductive Heat Transfer  thermal_type=foundation.enum.ConstantVariableTabulated.Constant  wall_geometry=foundation.enum.ConductionWallGeometry.Planar  area=8.86*3 m^2  thickness=0.01 m  d_in=0.05 m  d_out=0.1 m  L=1 m  th_cond_min=10 W/(K*m)  th_cond=k_concrete W/(K*m)  th_cond_TLU=[413, 401, 392, 383, 371, 357, 342] W/(K*m)  temp_TLU=[200, 273, 400, 600, 800, 1000, 1200] K  T_specify=on  T_priority=None  T=273.15+25 K  T_nominal_specify=off  T_nominal_value=1  T_nominal_unit=K  Q_specify=off  Q_priority=None  Q=0 W  Q_nominal_specify=off  Q_nominal_value=1  Q_nominal_unit=W
  ปูนฉาบใน2 : fl_lib/Thermal/Thermal Elements/Conductive Heat Transfer  thermal_type=foundation.enum.ConstantVariableTabulated.Constant  wall_geometry=foundation.enum.ConductionWallGeometry.Planar  area=8.51*3 m^2  thickness=0.01 m  d_in=0.05 m  d_out=0.1 m  L=1 m  th_cond_min=10 W/(K*m)  th_cond=k_concrete W/(K*m)  th_cond_TLU=[413, 401, 392, 383, 371, 357, 342] W/(K*m)  temp_TLU=[200, 273, 400, 600, 800, 1000, 1200] K  T_specify=on  T_priority=None  T=273.15+25 K  T_nominal_specify=off  T_nominal_value=1  T_nominal_unit=K  Q_specify=off  Q_priority=None  Q=0 W  Q_nominal_specify=off  Q_nominal_value=1  Q_nominal_unit=W
  ปูนฉาบใน3 : fl_lib/Thermal/Thermal Elements/Conductive Heat Transfer  thermal_type=foundation.enum.ConstantVariableTabulated.Constant  wall_geometry=foundation.enum.ConductionWallGeometry.Planar  area=8.86*3 m^2  thickness=0.01 m  d_in=0.05 m  d_out=0.1 m  L=1 m  th_cond_min=10 W/(K*m)  th_cond=k_concrete W/(K*m)  th_cond_TLU=[413, 401, 392, 383, 371, 357, 342] W/(K*m)  temp_TLU=[200, 273, 400, 600, 800, 1000, 1200] K  T_specify=on  T_priority=None  T=273.15+25 K  T_nominal_specify=off  T_nominal_value=1  T_nominal_unit=K  Q_specify=off  Q_priority=None  Q=0 W  Q_nominal_specify=off  Q_nominal_value=1  Q_nominal_unit=W
  อิฐมวลเบานอก : fl_lib/Thermal/Thermal Elements/Conductive Heat Transfer  thermal_type=foundation.enum.ConstantVariableTabulated.Constant  wall_geometry=foundation.enum.ConductionWallGeometry.Planar  area=8.51*3 m^2  thickness=0.05 m  d_in=0.05 m  d_out=0.1 m  L=1 m  th_cond_min=10 W/(K*m)  th_cond=k_Block W/(K*m)  th_cond_TLU=[413, 401, 392, 383, 371, 357, 342] W/(K*m)  temp_TLU=[200, 273, 400, 600, 800, 1000, 1200] K  T_specify=off  T_priority=None  T=0 K  T_nominal_specify=off  T_nominal_value=1  T_nominal_unit=K  Q_specify=off  Q_priority=None  Q=0 W  Q_nominal_specify=off  Q_nominal_value=1  Q_nominal_unit=W
  อิฐมวลเบานอก1 : fl_lib/Thermal/Thermal Elements/Conductive Heat Transfer  thermal_type=foundation.enum.ConstantVariableTabulated.Constant  wall_geometry=foundation.enum.ConductionWallGeometry.Planar  area=8.86*3 m^2  thickness=0.065 m  d_in=0.05 m  d_out=0.1 m  L=1 m  th_cond_min=10 W/(K*m)  th_cond=k_Block W/(K*m)  th_cond_TLU=[413, 401, 392, 383, 371, 357, 342] W/(K*m)  temp_TLU=[200, 273, 400, 600, 800, 1000, 1200] K  T_specify=off  T_priority=None  T=0 K  T_nominal_specify=off  T_nominal_value=1  T_nominal_unit=K  Q_specify=off  Q_priority=None  Q=0 W  Q_nominal_specify=off  Q_nominal_value=1  Q_nominal_unit=W
  อิฐมวลเบานอก2 : fl_lib/Thermal/Thermal Elements/Conductive Heat Transfer  thermal_type=foundation.enum.ConstantVariableTabulated.Constant  wall_geometry=foundation.enum.ConductionWallGeometry.Planar  area=8.51*3 m^2  thickness=0.065 m  d_in=0.05 m  d_out=0.1 m  L=1 m  th_cond_min=10 W/(K*m)  th_cond=k_Block W/(K*m)  th_cond_TLU=[413, 401, 392, 383, 371, 357, 342] W/(K*m)  temp_TLU=[200, 273, 400, 600, 800, 1000, 1200] K  T_specify=off  T_priority=None  T=0 K  T_nominal_specify=off  T_nominal_value=1  T_nominal_unit=K  Q_specify=off  Q_priority=None  Q=0 W  Q_nominal_specify=off  Q_nominal_value=1  Q_nominal_unit=W
  อิฐมวลเบานอก3 : fl_lib/Thermal/Thermal Elements/Conductive Heat Transfer  thermal_type=foundation.enum.ConstantVariableTabulated.Constant  wall_geometry=foundation.enum.ConductionWallGeometry.Planar  area=8.86*3 m^2  thickness=0.065 m  d_in=0.05 m  d_out=0.1 m  L=1 m  th_cond_min=10 W/(K*m)  th_cond=k_Block W/(K*m)  th_cond_TLU=[413, 401, 392, 383, 371, 357, 342] W/(K*m)  temp_TLU=[200, 273, 400, 600, 800, 1000, 1200] K  T_specify=off  T_priority=None  T=0 K  T_nominal_specify=off  T_nominal_value=1  T_nominal_unit=K  Q_specify=off  Q_priority=None  Q=0 W  Q_nominal_specify=off  Q_nominal_value=1  Q_nominal_unit=W
  อิฐมวลเบาใน : fl_lib/Thermal/Thermal Elements/Conductive Heat Transfer  thermal_type=foundation.enum.ConstantVariableTabulated.Constant  wall_geometry=foundation.enum.ConductionWallGeometry.Planar  area=8.51*3 m^2  thickness=0.05 m  d_in=0.05 m  d_out=0.1 m  L=1 m  th_cond_min=10 W/(K*m)  th_cond=k_Block W/(K*m)  th_cond_TLU=[413, 401, 392, 383, 371, 357, 342] W/(K*m)  temp_TLU=[200, 273, 400, 600, 800, 1000, 1200] K  T_specify=off  T_priority=None  T=0 K  T_nominal_specify=off  T_nominal_value=1  T_nominal_unit=K  Q_specify=off  Q_priority=None  Q=0 W  Q_nominal_specify=off  Q_nominal_value=1  Q_nominal_unit=W
  อิฐมวลเบาใน1 : fl_lib/Thermal/Thermal Elements/Conductive Heat Transfer  thermal_type=foundation.enum.ConstantVariableTabulated.Constant  wall_geometry=foundation.enum.ConductionWallGeometry.Planar  area=8.86*3 m^2  thickness=0.065 m  d_in=0.05 m  d_out=0.1 m  L=1 m  th_cond_min=10 W/(K*m)  th_cond=k_Block W/(K*m)  th_cond_TLU=[413, 401, 392, 383, 371, 357, 342] W/(K*m)  temp_TLU=[200, 273, 400, 600, 800, 1000, 1200] K  T_specify=on  T_priority=None  T=273.15+25 K  T_nominal_specify=off  T_nominal_value=1  T_nominal_unit=K  Q_specify=off  Q_priority=None  Q=0 W  Q_nominal_specify=off  Q_nominal_value=1  Q_nominal_unit=W
  อิฐมวลเบาใน2 : fl_lib/Thermal/Thermal Elements/Conductive Heat Transfer  thermal_type=foundation.enum.ConstantVariableTabulated.Constant  wall_geometry=foundation.enum.ConductionWallGeometry.Planar  area=8.51*3 m^2  thickness=0.065 m  d_in=0.05 m  d_out=0.1 m  L=1 m  th_cond_min=10 W/(K*m)  th_cond=k_Block W/(K*m)  th_cond_TLU=[413, 401, 392, 383, 371, 357, 342] W/(K*m)  temp_TLU=[200, 273, 400, 600, 800, 1000, 1200] K  T_specify=on  T_priority=None  T=273.15+25 K  T_nominal_specify=off  T_nominal_value=1  T_nominal_unit=K  Q_specify=off  Q_priority=None  Q=0 W  Q_nominal_specify=off  Q_nominal_value=1  Q_nominal_unit=W
  อิฐมวลเบาใน3 : fl_lib/Thermal/Thermal Elements/Conductive Heat Transfer  thermal_type=foundation.enum.ConstantVariableTabulated.Constant  wall_geometry=foundation.enum.ConductionWallGeometry.Planar  area=8.86*3 m^2  thickness=0.065 m  d_in=0.05 m  d_out=0.1 m  L=1 m  th_cond_min=10 W/(K*m)  th_cond=k_Block W/(K*m)  th_cond_TLU=[413, 401, 392, 383, 371, 357, 342] W/(K*m)  temp_TLU=[200, 273, 400, 600, 800, 1000, 1200] K  T_specify=on  T_priority=None  T=273.15+25 K  T_nominal_specify=off  T_nominal_value=1  T_nominal_unit=K  Q_specify=off  Q_priority=None  Q=0 W  Q_nominal_specify=off  Q_nominal_value=1  Q_nominal_unit=W
  tag scope: Envi=global, P1=global, P2=global, P3=global, P4=global, h1=global, h2=global, h3=global, h4=global
  wires:
  Constant/1 -> Simulink-PS Converter/1, [Envi]
  Constant1/1 -> Simulink-PS Converter1/1
  Constant2/1 -> Simulink-PS Converter2/1
  PS-Simulink Converter1/1 -> Scope1/2
  Mux1/1 -> P-H Diagram (2P)/1
  Mux2/1 -> P-H Diagram (2P)/2
  PS-Simulink Converter6/1 -> Display2/1
  PS-Simulink Converter/1 -> Scope/1, Display/1, error/1(Simualtion)  "simulation"
  [on_off] -> Scope/2, Simulink-PS Converter3/1
  [on_off] -> Scope/3
  PS-Simulink Converter7/1 -> Scope1/1  "evap"
  [on_off] -> Simulink-PS Converter4/1
  PS-Simulink Converter8/1 -> Display1/1
  Subsystem1/1(P) -> [P2]
  Subsystem1/2(h) -> [h2]
  Subsystem2/1(P) -> [P3]
  Subsystem2/2(h) -> [h3]
  [P2] -> Mux1/2
  [h2] -> Mux2/2
  [h3] -> Mux2/3
  [P3] -> Mux1/3
  Subsystem3/2(h) -> [h1]
  Subsystem3/1(P) -> [P1]
  [P1] -> Mux1/1
  [h1] -> Mux2/1
  Subsystem/1(P) -> [P4]
  Subsystem/2(h) -> [h4]
  [P4] -> Mux1/4
  [h4] -> Mux2/4
  Constant3/1 -> [on_off]
  connections:
  Simulink-PS Converter/RConn1 -- Controlled Temperature Source/RConn1
  Thermal Reference/LConn1 -- Controlled Temperature Source/RConn2
  ปูนฉาบนอก/LConn1 -- Convective Heat Transfer/RConn1
  ปูนฉาบใน/RConn1 -- Convective Heat Transfer1/LConn1
  Thermal Mass/LConn1 -- อิฐมวลเบาใน/LConn1 -- อิฐมวลเบานอก/RConn1
  Controlled Temperature Source/LConn1 -- Convective Heat Transfer6/LConn1 -- Convective Heat Transfer4/LConn1 -- Convective Heat Transfer2/LConn1 -- Convective Heat Transfer/LConn1
  Temperature Sensor/LConn1 -- Constant Volume Chamber (MA)2/RConn3 -- Heat Flow Rate Sensor/RConn2
  PS-Simulink Converter/LConn1 -- Temperature Sensor/RConn2
  Thermal Reference1/LConn1 -- Temperature Sensor/RConn1
  ปูนฉาบนอก/RConn1 -- อิฐมวลเบานอก/LConn1
  อิฐมวลเบาใน/RConn1 -- ปูนฉาบใน/LConn1
  Thermal Mass1/LConn1 -- อิฐมวลเบานอก1/RConn1 -- อิฐมวลเบาใน1/LConn1
  ปูนฉาบใน1/RConn1 -- Convective Heat Transfer3/LConn1
  ปูนฉาบนอก1/RConn1 -- อิฐมวลเบานอก1/LConn1
  ปูนฉาบนอก1/LConn1 -- Convective Heat Transfer2/RConn1
  อิฐมวลเบาใน1/RConn1 -- ปูนฉาบใน1/LConn1
  Thermal Mass2/LConn1 -- อิฐมวลเบานอก2/RConn1 -- อิฐมวลเบาใน2/LConn1
  ปูนฉาบนอก2/LConn1 -- Convective Heat Transfer4/RConn1
  อิฐมวลเบาใน2/RConn1 -- ปูนฉาบใน2/LConn1
  ปูนฉาบใน2/RConn1 -- Convective Heat Transfer5/LConn1
  ปูนฉาบนอก2/RConn1 -- อิฐมวลเบานอก2/LConn1
  Thermal Mass3/LConn1 -- อิฐมวลเบานอก3/RConn1 -- อิฐมวลเบาใน3/LConn1
  ปูนฉาบนอก3/RConn1 -- อิฐมวลเบานอก3/LConn1
  ปูนฉาบใน3/RConn1 -- Convective Heat Transfer7/LConn1
  ปูนฉาบนอก3/LConn1 -- Convective Heat Transfer6/RConn1
  อิฐมวลเบาใน3/RConn1 -- ปูนฉาบใน3/LConn1
  Thermal Reference2/LConn1 -- Labtop/RConn2
  Simulink-PS Converter1/RConn1 -- Labtop/RConn1
  Thermal Reference3/LConn1 -- People/RConn2
  Simulink-PS Converter2/RConn1 -- People/RConn1
  PS-Simulink Converter1/LConn1 -- Heat Flow Rate Sensor/RConn1
  Convective Heat Transfer7/RConn1 -- Heat Flow Rate Sensor/LConn1 -- Convective Heat Transfer1/RConn1 -- Labtop/LConn1 -- People/LConn1 -- Convective Heat Transfer3/RConn1 -- Convective Heat Transfer5/RConn1
  Evaporator (2P-MA)/RConn1 -- Flow Rate Sensor (MA)/RConn1
  Evaporator (2P-MA)/RConn2 -- Pipe (MA)1/RConn1
  Receiver Accumulator (2P)/RConn2 -- Thermostatic Expansion Valve (2P)/LConn1
  Pipe (MA)/LConn2 -- Perfect Insulator/LConn1
  Pipe (MA)/RConn1 -- Fan (MA)/LConn1
  Pipe (MA)/LConn1 -- Constant Volume Chamber (MA)2/LConn1
  Pipe (MA)1/LConn1 -- Constant Volume Chamber (MA)2/LConn2
  Pipe (MA)1/LConn2 -- Perfect Insulator1/LConn1
  Fan (MA)/RConn2 -- Ideal Angular Velocity Source/LConn1 -- Mechanical Rotational Reference/LConn1
  Ideal Angular Velocity Source/RConn2 -- Fan (MA)/LConn2
  Ideal Angular Velocity Source/RConn1 -- PS Gain/RConn1
  Flow Rate Sensor (MA)/LConn1 -- Moist Air Properties (MA)1/RConn1 -- Fan (MA)/RConn1
  PS-Simulink Converter6/LConn1 -- Flow Rate Sensor (MA)/RConn2
  Simulink-PS Converter3/RConn1 -- PS Gain/LConn1
  Evaporator (2P-MA)/LConn3 -- PS-Simulink Converter7/LConn1
  Positive-Displacement Compressor (2P)/LConn1 -- Solver Configuration1/RConn1 -- Two-Phase Fluid Predefined Properties (2P)/RConn1 -- Thermostatic Expansion Valve (2P)/LConn2 -- Subsystem3/LConn1 -- Evaporator (2P-MA)/LConn2
  Mechanical Rotational Reference1/LConn1 -- Ideal Angular Velocity Source1/RConn2 -- Positive-Displacement Compressor (2P)/LConn2
  Flow Rate Sensor (2P)/LConn1 -- Positive-Displacement Compressor (2P)/RConn1 -- Subsystem1/LConn1
  Condenser/LConn2 -- Receiver Accumulator (2P)/LConn2 -- Subsystem2/LConn1
  Flow Rate Sensor (2P)/RConn1 -- Condenser/LConn1
  Simulink-PS Converter4/RConn1 -- PS Gain1/LConn1
  Ideal Angular Velocity Source1/LConn1 -- Positive-Displacement Compressor (2P)/RConn2
  PS-Simulink Converter8/LConn1 -- Flow Rate Sensor (2P)/RConn2
  PS Gain1/RConn1 -- Ideal Angular Velocity Source1/RConn1
  Reservoir (MA)/LConn1 -- Condenser/RConn2
  Reservoir (MA)1/LConn1 -- Flow Rate Source (MA)/LConn1
  Flow Rate Source (MA)/RConn1 -- Condenser/RConn1
  Thermostatic Expansion Valve (2P)/RConn1 -- Subsystem/LConn1 -- Evaporator (2P-MA)/LConn1
